simulink model "hexMotorModel"  (R2024a)
settings: configuration reference "autoCodeSILConfigurationParams" (kept outside this file)
undefined symbols (not defined in the file): actuatorDelay_s, airDensityAtStd_kgpm3, rpm2radps, stepSize_s, vehicleParams
libraries: matrix_library x1
settings Model: Creator=jerem  LastModifiedBy=jerem
settings ConfigSetRef: SourceName=autoCodeSILConfigurationParams  SourceLocation=Base Workspace

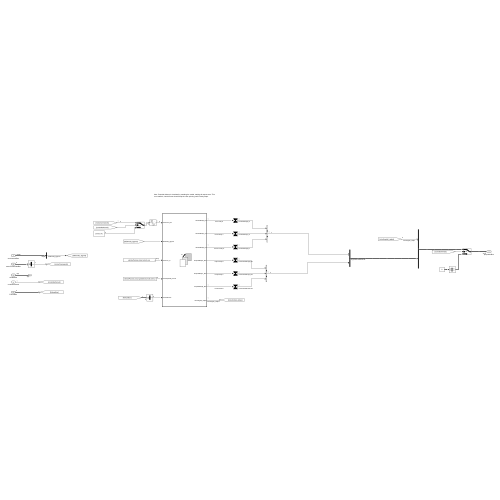
[thumbnail: Simulink's stored preview of the top-level diagram]
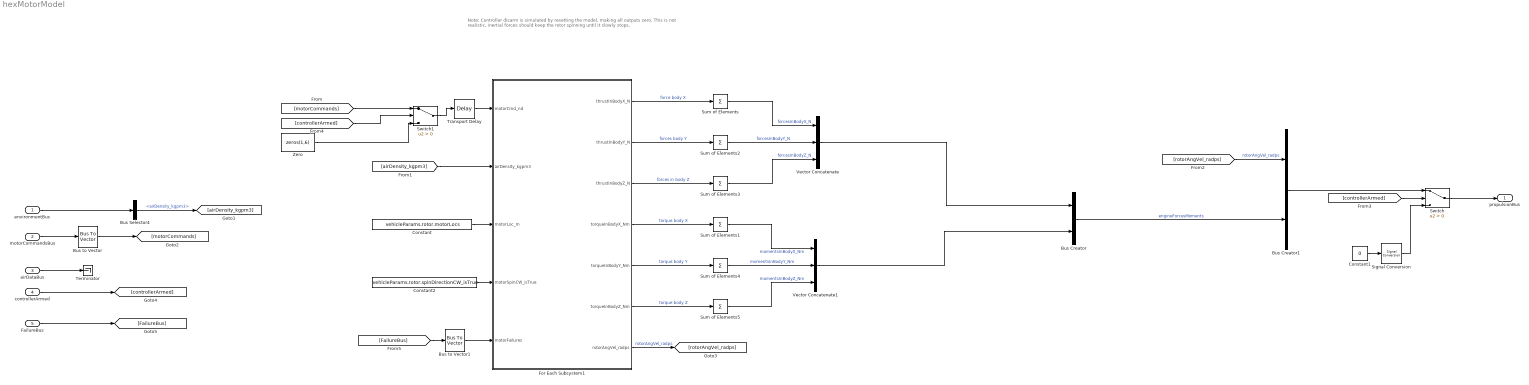
== system hexMotorModel ==
  note: Note: Controller disarm is simulated by resetting the model, making all outputs zero. This is not realistic, inertial forces should keep the rotor spinning until it slowly stops.
  environmentBus : Inport  OutDataTypeStr=Bus: EnvironmentBus
  motorCommandsBus : Inport  Port=2  OutDataTypeStr=Bus: MotorCommandHexBus
  airDataBus : Inport  Port=3  OutDataTypeStr=Bus: AirDataBus  SampleTime=stepSize_s
  controllerArmed : Inport  Port=4
  FailureBus : Inport  Port=5  OutDataTypeStr=Bus: FailureBus
  Bus Creator : BusCreator  Inputs=2  OutDataTypeStr=Bus: ComponentForcesMomentsBus  NonVirtualBus=on
      settings: InheritFromInputs=off
  Bus Creator1 : BusCreator  Inputs=2  OutDataTypeStr=Bus: PropulsionBus  NonVirtualBus=on
  Bus Selector4 : BusSelector  OutputSignals=AirEnvironment.airDensity_kgpm3
  Bus to Vector : BusToVector
  Bus to Vector1 : BusToVector
  Constant : Constant  Value=vehicleParams.rotor.motorLocs  SampleTime=stepSize_s
  Constant1 : Constant  Value=0  OutDataTypeStr=Bus: PropulsionBus  SampleTime=stepSize_s
  Constant2 : Constant  Value=vehicleParams.rotor.spinDirectionCW_isTrue  SampleTime=stepSize_s
  For Each Subsystem1 : Subsystem  TreatAsAtomicUnit=on
  Signal Conversion : SignalConversion  ConversionOutput=Nonvirtual bus  OverrideOpt=off
  Sum of Elements{,1..5} (6 alike) : Sum  Inputs=+
  Switch : Switch  Criteria=u2 > Threshold  SaturateOnIntegerOverflow=off  InputSameDT=off
  Switch1 : Switch  Criteria=u2 > Threshold  SaturateOnIntegerOverflow=off  InputSameDT=off
  Terminator : Terminator
  Transport Delay : TransportDelay  DelayTime=actuatorDelay_s
  Vector Concatenate : Concatenate  NumInputs=3
  Vector Concatenate1 : Concatenate  NumInputs=3
  Zero : Constant  Value=zeros(1,6)  OutDataTypeStr=Inherit: Inherit via back propagation  SampleTime=stepSize_s
  propulsionBus : Outport  OutDataTypeStr=Bus: PropulsionBus
  wires:
  environmentBus/1 -> Bus Selector4/1
  For Each Subsystem1/1(thrustInBodyX_N) -> Sum of Elements/1  "force body X"
  For Each Subsystem1/4(torqueInBodyX_Nm) -> Sum of Elements1/1  "torque body X"
  Constant/1 -> For Each Subsystem1/3(motorLoc_m)
  Bus Selector4/1 -> [airDensity_kgpm3]  "<airDensity_kgpm3>"
  [airDensity_kgpm3] -> For Each Subsystem1/2(airDensity_kgpm3)
  motorCommandsBus/1 -> Bus to Vector/1
  For Each Subsystem1/7(rotorAngVel_radps) -> [rotorAngVel_radps]  "rotorAngVel_radps"
  [rotorAngVel_radps] -> Bus Creator1/1  "rotorAngVel_radps"
  Bus Creator/1 -> Bus Creator1/2  "engineForcesMoments"
  Bus to Vector/1 -> [motorCommands]
  For Each Subsystem1/2(thrustInBodyY_N) -> Sum of Elements2/1  "forces body Y"
  For Each Subsystem1/3(thrustInBodyZ_N) -> Sum of Elements3/1  "forces in body Z"
  Sum of Elements/1 -> Vector Concatenate/1  "forcesInBodyX_N"
  Sum of Elements2/1 -> Vector Concatenate/2  "forcesInBodyY_N"
  Sum of Elements3/1 -> Vector Concatenate/3  "forcesInBodyZ_N"
  For Each Subsystem1/5(torqueInBodyY_Nm) -> Sum of Elements4/1  "torque body Y"
  For Each Subsystem1/6(torqueInBodyZ_Nm) -> Sum of Elements5/1  "torque body Z"
  Sum of Elements4/1 -> Vector Concatenate1/2  "momentsInBodyY_Nm"
  Sum of Elements1/1 -> Vector Concatenate1/1  "momentsInBodyX_Nm"
  Sum of Elements5/1 -> Vector Concatenate1/3  "momentsInBodyZ_Nm"
  airDataBus/1 -> Terminator/1
  Vector Concatenate1/1 -> Bus Creator/2
  Vector Concatenate/1 -> Bus Creator/1
  controllerArmed/1 -> [controllerArmed]
  Switch/1 -> propulsionBus/1
  Bus Creator1/1 -> Switch/1
  [controllerArmed] -> Switch/2
  Constant1/1 -> Signal Conversion/1
  Signal Conversion/1 -> Switch/3
  Switch1/1 -> Transport Delay/1
  [motorCommands] -> Switch1/1
  [controllerArmed] -> Switch1/2
  Zero/1 -> Switch1/3
  Constant2/1 -> For Each Subsystem1/4(motorSpinCW_isTrue)
  Transport Delay/1 -> For Each Subsystem1/1(motorCmd_nd)
  FailureBus/1 -> [FailureBus]
  [FailureBus] -> Bus to Vector1/1
  Bus to Vector1/1 -> For Each Subsystem1/5(motorFailures)

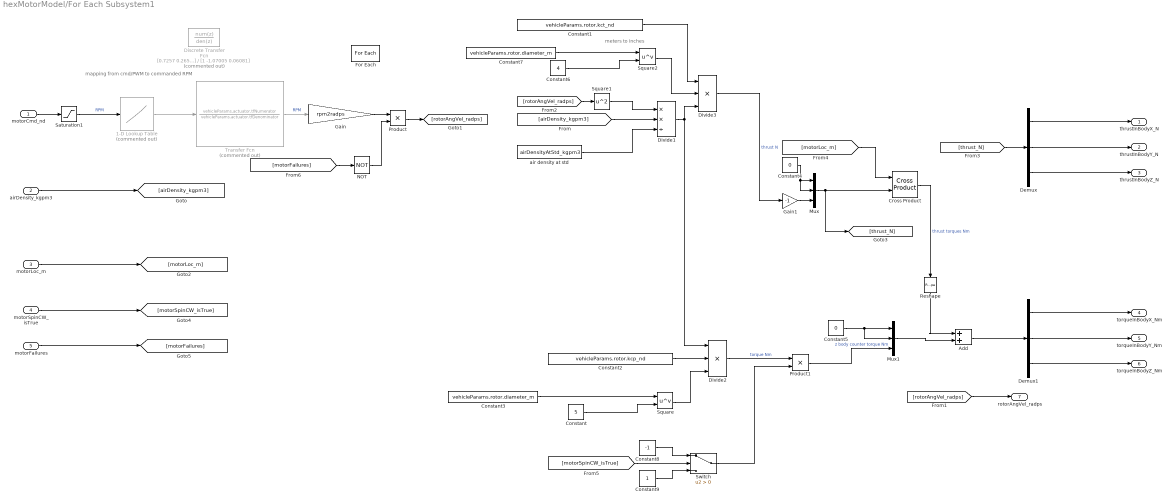
== system hexMotorModel/For Each Subsystem1 ==
  note: meters to inches
  note: mapping from cmd/PWM to commanded RPM
  motorCmd_nd : Inport  Partition=on  PartitionDimension=1  PartitionWidth=1  PartitionOffset=0
  airDensity_kgpm3 : Inport  Port=2
  motorLoc_m : Inport  Port=3  Partition=on  PartitionDimension=1  PartitionWidth=1  PartitionOffset=0
  motorSpinCW_isTrue : Inport  Port=4  Partition=on  PartitionDimension=1  PartitionWidth=1  PartitionOffset=0
  motorFailures : Inport  Port=5  Partition=on  PartitionDimension=1  PartitionWidth=1  PartitionOffset=0
  1-D Lookup Table : Lookup_n-D  Commented=on  NumberOfTableDimensions=1  BreakpointsForDimension1=vehicleParams.rotor.cmdToRpmBkpts_nd  Table=vehicleParams.rotor.cmdToRpmData  RemoveProtectionInput=on  InternalRulePriority=Speed  RndMeth=Simplest
  Add : Sum
  Constant : Constant  Value=5  SampleTime=stepSize_s
  Constant1 : Constant  Value=vehicleParams.rotor.kct_nd  SampleTime=stepSize_s
  Constant2 : Constant  Value=vehicleParams.rotor.kcp_nd  SampleTime=stepSize_s
  Constant3 : Constant  Value=vehicleParams.rotor.diameter_m  SampleTime=stepSize_s
  Constant4 : Constant  Value=0  SampleTime=stepSize_s
  Constant5 : Constant  Value=0  SampleTime=stepSize_s
  Constant6 : Constant  Value=4  SampleTime=stepSize_s
  Constant7 : Constant  Value=vehicleParams.rotor.diameter_m  SampleTime=stepSize_s
  Constant8 : Constant  Value=-1  SampleTime=stepSize_s
  Constant9 : Constant  SampleTime=stepSize_s
  Cross Product : matrix_library/Cross Product
  Demux : Demux  Outputs=3
  Demux1 : Demux  Outputs=3
  Discrete Transfer Fcn : DiscreteTransferFcn  Commented=on  Numerator=[0.7257 0.265]  Denominator=[1 -1.07005 0.06081]
  Divide1 : Product  Inputs=**/
  Divide2 : Product  Inputs=***
  Divide3 : Product  Inputs=***
  For Each : ForEach  DisableCoverage=on
  Gain : Gain  Gain=rpm2radps
  Gain1 : Gain  Gain=-1
  Mux : Mux  Inputs=3
  Mux1 : Mux  Inputs=3
  NOT : Logic  Operator=NOT  IconShape=distinctive  AllPortsSameDT=off  OutDataTypeStr=boolean
  Product : Product
  Product1 : Product
  Reshape : Reshape
  Saturation1 : Saturate  UpperLimit=1  LowerLimit=0
  Square : Math  Operator=pow
  Square1 : Math  Operator=square
  Square2 : Math  Operator=pow
  Switch : Switch  Criteria=u2 > Threshold  SaturateOnIntegerOverflow=off  InputSameDT=off
  Transfer Fcn : TransferFcn  Commented=on  Numerator=vehicleParams.actuator.tfNumerator  Denominator=vehicleParams.actuator.tfDenominator
  air density at std : Constant  Value=airDensityAtStd_kgpm3  SampleTime=stepSize_s
  thrustInBodyX_N : Outport  ConcatenationDimension=1
  thrustInBodyY_N : Outport  Port=2  ConcatenationDimension=1
  thrustInBodyZ_N : Outport  Port=3  ConcatenationDimension=1
  torqueInBodyX_Nm : Outport  Port=4  ConcatenationDimension=1
  torqueInBodyY_Nm : Outport  Port=5  ConcatenationDimension=1
  torqueInBodyZ_Nm : Outport  Port=6  ConcatenationDimension=1
  rotorAngVel_radps : Outport  Port=7  ConcatenationDimension=1
  wires:
  Saturation1/1 -> 1-D Lookup Table/1  "RPM"
  Divide1/1 -> Divide2/1, Divide3/3
  Constant1/1 -> Divide3/1
  airDensity_kgpm3/1 -> [airDensity_kgpm3]
  [rotorAngVel_radps] -> Square1/1
  Constant4/1 -> Mux/1, Mux/2
  Mux/1 -> [thrust_N], Cross Product/2
  Cross Product/1 -> Reshape/1  "thrust torques Nm"
  motorLoc_m/1 -> [motorLoc_m]
  Product1/1 -> Mux1/3  "z body counter torque Nm"
  Constant5/1 -> Mux1/1, Mux1/2
  Mux1/1 -> Add/2
  Square1/1 -> Divide1/1
  [airDensity_kgpm3] -> Divide1/2
  air density at std/1 -> Divide1/3
  Divide3/1 -> Gain1/1  "thrust N"
  Constant2/1 -> Divide2/2
  Divide2/1 -> Product1/1  "torque Nm"
  [rotorAngVel_radps] -> rotorAngVel_radps/1
  motorCmd_nd/1 -> Saturation1/1
  Constant/1 -> Square/2
  Square/1 -> Divide2/3
  Constant6/1 -> Square2/2
  Square2/1 -> Divide3/2
  [motorLoc_m] -> Cross Product/1
  Reshape/1 -> Add/1
  [thrust_N] -> Demux/1
  Demux/1 -> thrustInBodyX_N/1
  Demux/2 -> thrustInBodyY_N/1
  Demux/3 -> thrustInBodyZ_N/1
  Add/1 -> Demux1/1
  Demux1/1 -> torqueInBodyX_Nm/1
  Demux1/2 -> torqueInBodyY_Nm/1
  Demux1/3 -> torqueInBodyZ_Nm/1
  motorSpinCW_isTrue/1 -> [motorSpinCW_isTrue]
  [motorSpinCW_isTrue] -> Switch/2
  Constant8/1 -> Switch/1
  Constant9/1 -> Switch/3
  Switch/1 -> Product1/2
  Gain1/1 -> Mux/3
  Constant7/1 -> Square2/1
  Constant3/1 -> Square/1
  motorFailures/1 -> [motorFailures]
  [motorFailures] -> NOT/1
  Gain/1 -> Product/1
  NOT/1 -> Product/2
  Product/1 -> [rotorAngVel_radps]
  Transfer Fcn/1 -> Gain/1  "RPM"
  1-D Lookup Table/1 -> Transfer Fcn/1
